simulink model "io_meta_info"  (Simulink 10.1)
settings: Solver=FixedStepDiscrete  StartTime=0.0  StopTime=10.0  RelTol=1e-3  EnableMultiTasking=on
settings Model: Creator=Demo  LastModifiedBy=MaximeBe
settings DataIOCC: LimitDataPoints=on  SaveFormat=Dataset
settings OptimizationCC: ZeroExternalMemoryAtStartup=off  ZeroInternalMemoryAtStartup=off  LifeSpan=auto
settings DebuggingCC: UnderspecifiedInitializationDetection=Simplified  MergeDetectMultiDrivingBlocksExec=error  AllowSymbolicDim=off  SFExecutionAtInitializationDiag=warning
settings HardwareCC: ProdBitPerPointer=64  ProdBitPerSizeT=64  ProdBitPerPtrDiffT=64  ProdLargestAtomicFloat=Float  ProdIntDivRoundTo=Zero  ProdEndianess=LittleEndian  ProdWordSize=64  ProdHWDeviceType=Intel->x86-64 (Windows64)
settings RTWCC: Description=Generate an RTMaps component embedding the model  SystemTargetFile=rtmaps.tlc  TemplateMakefile=rtmaps_default_tmf  PostCodeGenCommand=rtmaps_post_code_generation(buildInfo)  RetainRTWFile=on  TargetLang=C++
settings STFCustomTargetCC: ModelReferenceCompliant=off  ConcurrentExecutionCompliant=on  CombineOutputUpdateFcns=on  MultiInstanceERTCode=on  CodeInterfacePackaging=C++ class  CPPClassGenCompliant=on  GRTInterface=off  SystemTargetFile=rtmaps.tlc
settings GRTTargetCC: ModelReferenceCompliant=off  ParMdlRefBuildCompliant=off  CompOptLevelCompliant=off  CombineOutputUpdateFcns=on  MatFileLogging=off  MultiInstanceERTCode=on  CodeInterfacePackaging=C++ class  GRTInterface=off  UseToolchainInfoCompliant=off
settings CPPComponent: GenerateDestructor=on  ExternalIOMemberVisibility=private  GenerateExternalIOAccessMethods=Inlined structure-based method  ParameterMemberVisibility=public  InternalMemberVisibility=private  GenerateParameterAccessMethods=None  GenerateInternalMemberAccessMethods=None  UseOperatorNewForModelRefRegistration=off  IncludeModelTypesInModelClass=on

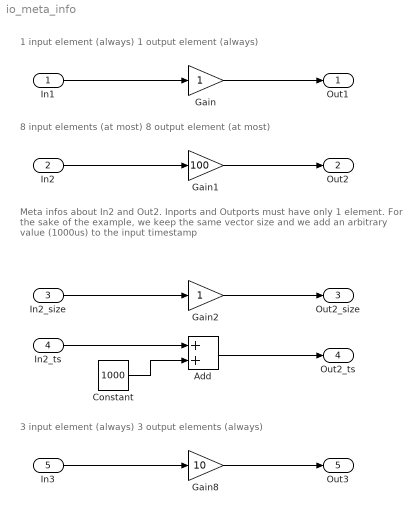
== system io_meta_info ==
  note: Meta infos about In2 and Out2.
      | Inports and Outports must have only 1 element.
      | For the sake of the example, we keep the same vector size
      | and we add an arbitrary value (1000us) to the input timestamp
  note: 3 input element (always)
      | 3 output elements (always)
  note: 8 input elements (at most)
      | 8 output element (at most)
  note: 1 input element (always)
      | 1 output element (always)
  In1 : Inport  OutDataTypeStr=double
  In2 : Inport  Port=2  OutDataTypeStr=uint32  PortDimensions=8
  In2_size : Inport  Port=3  OutDataTypeStr=int32
  In2_ts : Inport  Port=4  OutDataTypeStr=int32
  In3 : Inport  Port=5  OutDataTypeStr=single  PortDimensions=3
  Add : Sum
  Constant : Constant  Value=1000  OutDataTypeStr=int32
  Gain : Gain  OutDataTypeStr=double
  Gain1 : Gain  Gain=100  OutDataTypeStr=uint32
  Gain2 : Gain  OutDataTypeStr=int32
  Gain8 : Gain  Gain=10  OutDataTypeStr=single
  "Out1 " : Outport  OutDataTypeStr=double
  Out2 : Outport  Port=2  OutDataTypeStr=uint32
  Out2_size : Outport  Port=3  OutDataTypeStr=int32
  Out2_ts : Outport  Port=4  OutDataTypeStr=int32
  Out3 : Outport  Port=5  OutDataTypeStr=single
  wires:
  Gain/1 -> "Out1 "/1
  In1/1 -> Gain/1
  In2/1 -> Gain1/1
  Gain1/1 -> Out2/1
  Gain2/1 -> Out2_size/1
  In2_size/1 -> Gain2/1
  Add/1 -> Out2_ts/1
  Gain8/1 -> Out3/1
  In3/1 -> Gain8/1
  Constant/1 -> Add/2
  In2_ts/1 -> Add/1
